simulink model "sfun_keyboard_input_v1_2"  (Simulink 8.5)
settings: Solver=ode45  StartTime=0.0  StopTime=Inf  RelTol=1e-3
settings Model: Creator=pit  LastModifiedBy=Cecilia Ruiz Romero  CovSFcnEnable=off
settings OptimizationCC: InitFltsAndDblsToZero=on
settings DebuggingCC: SolverPrmCheckMsg=warning  FcnCallInpInsideContextMsg=UseLocalSettings

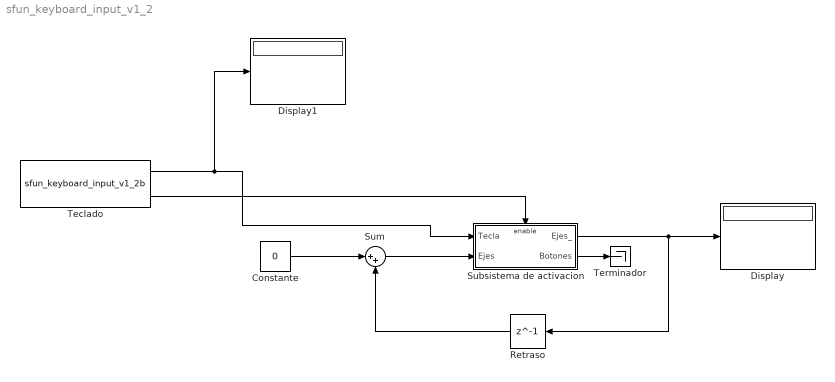
== system sfun_keyboard_input_v1_2 ==
  Constante : Constant  Value=0
  Display : Display
  Display1 : Display
  Retraso : Delay  DelayLength=1  InitialCondition=0  SampleTime=1e-16
  Subsistema de activacion : Subsystem  TreatAsAtomicUnit=on
  Sum : Sum  Inputs=|++
  Teclado : M-S-Function  FunctionName=sfun_keyboard_input_v1_2b  mask(Keyboard Input){}
      mask help: Keyboard Input
      mask Display: fprintf('Keyboard');
  Terminador : Terminator
  wires:
  Constante/1 -> Sum/1
  Sum/1 -> Subsistema de activacion/2(Ejes)
  Teclado/1 -> Display1/1, Subsistema de activacion/1(Tecla)
  Teclado/2 -> Subsistema de activacion/Enable
  Subsistema de activacion/1(Ejes_) -> Retraso/1, Display/1
  Retraso/1 -> Sum/2
  Subsistema de activacion/2(Botones) -> Terminador/1

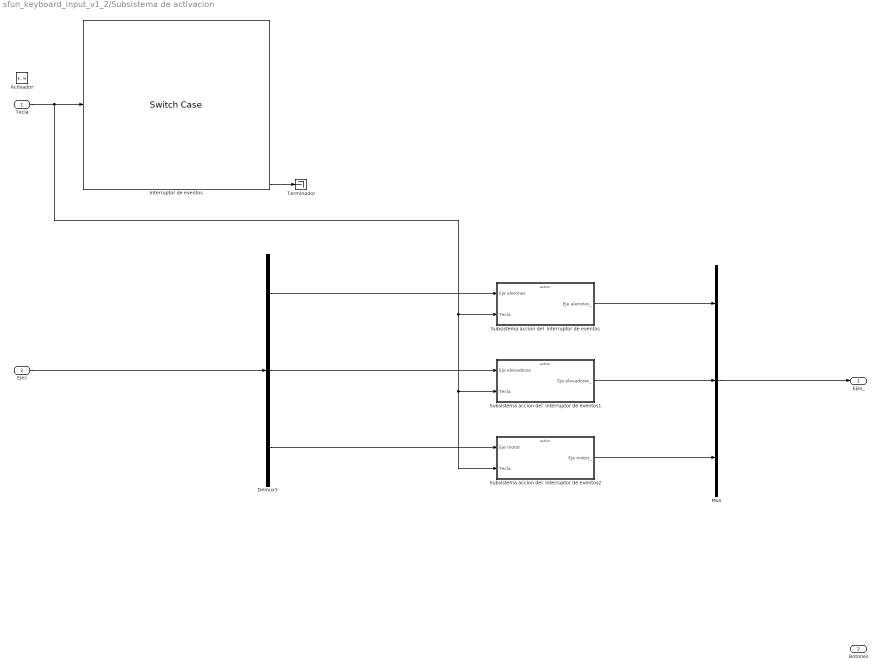
== system sfun_keyboard_input_v1_2/Subsistema de activacion ==
  Tecla : Inport
  Ejes : Inport  Port=2
  Activador : EnablePort
  Demux3 : Demux  Outputs=3
  Interruptor de eventos : SwitchCase  CaseConditions={48,49,50,51,52,53,54,[97,100],[115,119],[102,114]}
  Mux : Mux  Inputs=3
  Subsistema accion del  interruptor de eventos : Subsystem  TreatAsAtomicUnit=on
  Subsistema accion del  interruptor de eventos1 : Subsystem  TreatAsAtomicUnit=on
  Subsistema accion del  interruptor de eventos2 : Subsystem  TreatAsAtomicUnit=on
  Terminador : Terminator
  Ejes_ : Outport
  Botones : Outport  Port=2
  wires:
  Tecla/1 -> Subsistema accion del  interruptor de eventos/2(Tecla), Subsistema accion del  interruptor de eventos2/2(Tecla), Subsistema accion del  interruptor de eventos1/2(Tecla), Interruptor de eventos/1
  Ejes/1 -> Demux3/1
  Interruptor de eventos/11 -> Terminador/1
  Demux3/2 -> Subsistema accion del  interruptor de eventos1/1(Eje elevadores)
  Subsistema accion del  interruptor de eventos1/1(Eje elevadores_) -> Mux/2
  Demux3/1 -> Subsistema accion del  interruptor de eventos/1(Eje alerones)
  Demux3/3 -> Subsistema accion del  interruptor de eventos2/1(Eje motor)
  Subsistema accion del  interruptor de eventos/1(Eje alerones_) -> Mux/1
  Subsistema accion del  interruptor de eventos2/1(Eje motor_) -> Mux/3
  Mux/1 -> Ejes_/1

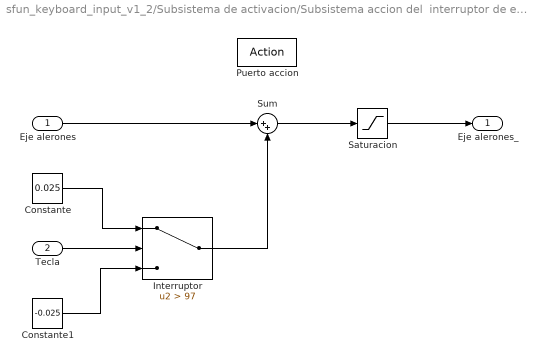
== system sfun_keyboard_input_v1_2/Subsistema de activacion/Subsistema accion del  interruptor de eventos ==
  Eje alerones : Inport
  Tecla : Inport  Port=2
  Puerto accion : ActionPort
  Constante : Constant  Value=0.025
  Constante1 : Constant  Value=-0.025
  Interruptor : Switch  Criteria=u2 > Threshold  Threshold=97
  Saturacion : Saturate  UpperLimit=1  LowerLimit=-1
  Sum : Sum  Inputs=|++
  Eje alerones_ : Outport
  wires:
  Tecla/1 -> Interruptor/2
  Constante1/1 -> Interruptor/3
  Constante/1 -> Interruptor/1
  Eje alerones/1 -> Sum/1
  Interruptor/1 -> Sum/2
  Sum/1 -> Saturacion/1
  Saturacion/1 -> Eje alerones_/1

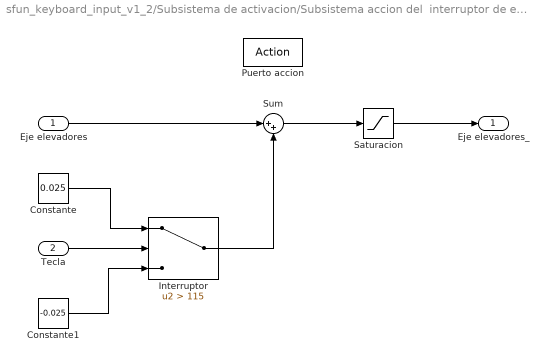
== system sfun_keyboard_input_v1_2/Subsistema de activacion/Subsistema accion del  interruptor de eventos1 ==
  Eje elevadores : Inport
  Tecla : Inport  Port=2
  Puerto accion : ActionPort
  Constante : Constant  Value=0.025
  Constante1 : Constant  Value=-0.025
  Interruptor : Switch  Criteria=u2 > Threshold  Threshold=115
  Saturacion : Saturate  UpperLimit=1  LowerLimit=-1
  Sum : Sum  Inputs=|++
  Eje elevadores_ : Outport
  wires:
  Eje elevadores/1 -> Sum/1
  Interruptor/1 -> Sum/2
  Sum/1 -> Saturacion/1
  Saturacion/1 -> Eje elevadores_/1
  Tecla/1 -> Interruptor/2
  Constante/1 -> Interruptor/1
  Constante1/1 -> Interruptor/3

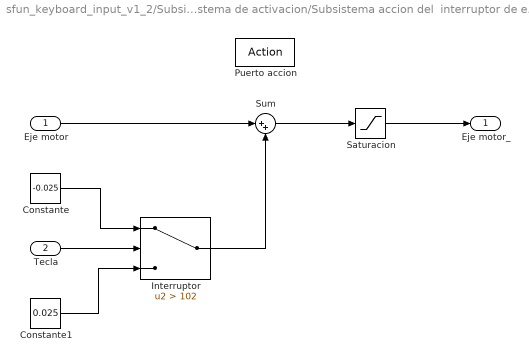
== system sfun_keyboard_input_v1_2/Subsistema de activacion/Subsistema accion del  interruptor de eventos2 ==
  Eje motor : Inport
  Tecla : Inport  Port=2
  Puerto accion : ActionPort
  Constante : Constant  Value=-0.025
  Constante1 : Constant  Value=0.025
  Interruptor : Switch  Criteria=u2 > Threshold  Threshold=102
  Saturacion : Saturate  UpperLimit=1  LowerLimit=-1
  Sum : Sum  Inputs=|++
  Eje motor_ : Outport
  wires:
  Tecla/1 -> Interruptor/2
  Eje motor/1 -> Sum/1
  Interruptor/1 -> Sum/2
  Sum/1 -> Saturacion/1
  Saturacion/1 -> Eje motor_/1
  Constante1/1 -> Interruptor/3
  Constante/1 -> Interruptor/1
